simulink model "LQR_finished"  (R2018b)
settings: Solver=VariableStepAuto  StartTime=0.0  StopTime=25  MinStep=1e-100  RelTol=1e-3
model workspace (MAT data in the model file):
  Af = 0.027
  Cd = 32.3127
  Q = 1
  R = 1
  Rx = 1.6517
  Tf = 25
  g = 9.81
  height = 0.12
  m = 3
  rho = 1.225
  v = 0
  width = 0.25
values from neighbouring files (symbols this model uses):
  K = lqr(A,B,100,1)    [lab6.m]
  p = 1.225    [lab6.m]
settings Model: Creator=vallon2  LastModifiedBy=Sunny
settings SFSimCC: SimUseLocalCustomCode=off
settings RTWCC: RTWUseLocalCustomCode=off

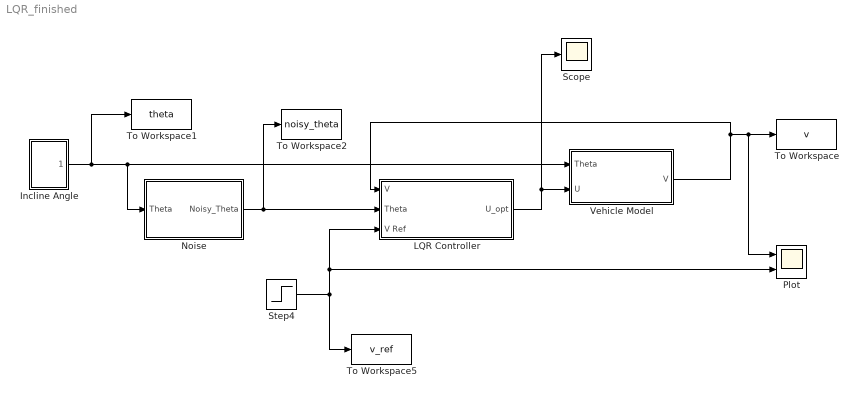
== system LQR_finished ==
  Incline Angle : Subsystem
  LQR Controller : Subsystem
  "Noise " : Subsystem
  "Plot " : Scope  NumInputPorts=2
  Scope : Scope
  Step4 : Step  Time=10  Before=0.5  SampleTime=0
  To Workspace : ToWorkspace  VariableName=v  SaveFormat=Timeseries  SampleTime=-1
  To Workspace1 : ToWorkspace  VariableName=theta  SaveFormat=Timeseries  SampleTime=-1
  To Workspace2 : ToWorkspace  VariableName=noisy_theta  SaveFormat=Timeseries  SampleTime=-1
  To Workspace5 : ToWorkspace  VariableName=v_ref  SaveFormat=Timeseries  SampleTime=-1
  Vehicle Model : Subsystem
  wires:
  Step4/1 -> To Workspace5/1, "Plot "/2, LQR Controller/3(V Ref)
  Vehicle Model/1(V) -> To Workspace/1, "Plot "/1, LQR Controller/1("V ")
  LQR Controller/1("U_opt ") -> Scope/1, Vehicle Model/2(U)
  "Noise "/1("Noisy_Theta ") -> LQR Controller/2(Theta), To Workspace2/1
  Incline Angle/1("Theta ") -> To Workspace1/1, Vehicle Model/1(Theta), "Noise "/1("Theta ")

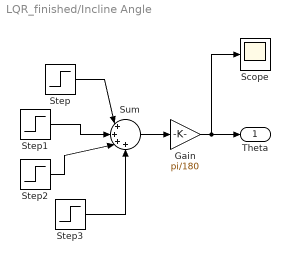
== system LQR_finished/Incline Angle ==
  Gain : Gain  Gain=pi/180
  Scope : Scope
  Step : Step  Time=3  After=10  SampleTime=0
  Step1 : Step  Time=8  After=10  SampleTime=0
  Step2 : Step  Time=13  After=-35  SampleTime=0
  Step3 : Step  Time=17  After=15  SampleTime=0
  Sum : Sum  Inputs=|++++
  "Theta " : Outport
  wires:
  Step/1 -> Sum/1
  Step1/1 -> Sum/2
  Step3/1 -> Sum/4
  Sum/1 -> Gain/1
  Gain/1 -> Scope/1, "Theta "/1
  Step2/1 -> Sum/3

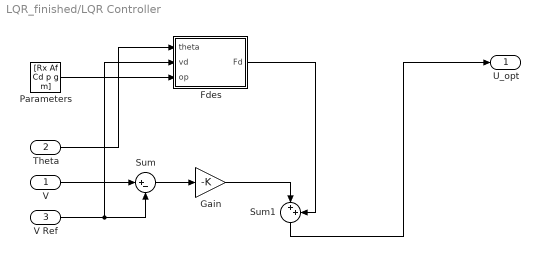
== system LQR_finished/LQR Controller ==
  "V " : Inport
  Theta : Inport  Port=2
  V Ref : Inport  Port=3
  Fdes : MATLAB Function  TreatAsAtomicUnit=on
  Gain : Gain  Gain=-K
  Parameters : Constant  Value=[Rx Af Cd p g m]
  Sum : Sum  Inputs=|+-
  Sum1 : Sum  Inputs=|++
  "U_opt " : Outport
  wires:
  "V "/1 -> Sum/1
  V Ref/1 -> Sum/2, Fdes/2(vd)
  Sum/1 -> Gain/1
  Fdes/1(Fd) -> Sum1/2
  Theta/1 -> Fdes/1(theta)
  Gain/1 -> Sum1/1
  Sum1/1 -> "U_opt "/1
  Parameters/1 -> Fdes/3(op)

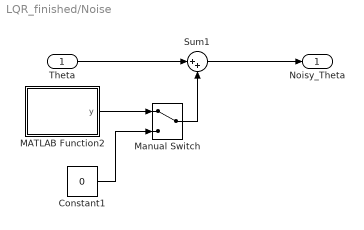
== system LQR_finished/Noise  ==
  "Theta " : Inport
  Constant1 : Constant  Value=0
  MATLAB Function2 : MATLAB Function  TreatAsAtomicUnit=on
  Manual Switch : ManualSwitch
  Sum1 : Sum  Inputs=|++
  "Noisy_Theta " : Outport
  wires:
  Constant1/1 -> Manual Switch/2
  Sum1/1 -> "Noisy_Theta "/1
  MATLAB Function2/1(y) -> Manual Switch/1
  "Theta "/1 -> Sum1/1
  Manual Switch/1 -> Sum1/2

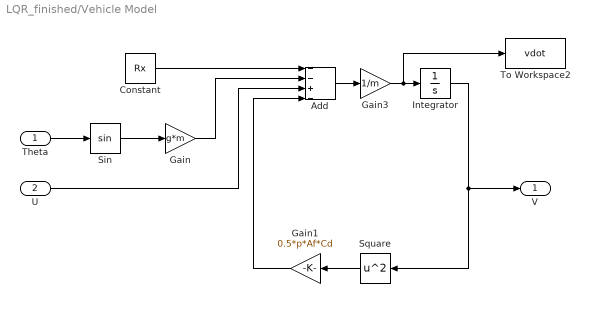
== system LQR_finished/Vehicle Model ==
  Theta : Inport
  U : Inport  Port=2
  Add : Sum  Inputs=--+-
  Constant : Constant  Value=Rx
  Gain : Gain  Gain=g*m
  Gain1 : Gain  Gain=0.5*p*Af*Cd
  Gain3 : Gain  Gain=1/m
  Integrator : Integrator
  Sin : Trigonometry
  Square : Math  Operator=square  SaturateOnIntegerOverflow=on
  To Workspace2 : ToWorkspace  VariableName=vdot  SaveFormat=Timeseries  SampleTime=-1
  V : Outport
  wires:
  Constant/1 -> Add/1
  Theta/1 -> Sin/1
  Sin/1 -> Gain/1
  Gain/1 -> Add/2
  U/1 -> Add/3
  Add/1 -> Gain3/1
  Square/1 -> Gain1/1
  Gain1/1 -> Add/4
  Integrator/1 -> Square/1, V/1
  Gain3/1 -> To Workspace2/1, Integrator/1

== matlab function LQR_finished/LQR Controller/Fdes ==
  data: theta input; Fd output; vd input; op input
function Fd = fcn( theta, vd, op)
Rx = op(1);
Af = op(2);
Cd = op(3);
p = op(4);
g = op(5);
m = op(6);
Fd = Rx+m*g*sin(theta)+0.5*p*Af*Cd*vd^2;

== matlab function LQR_finished/Noise /MATLAB Function2 ==
  data: y output
function y = noise
y = 0.01*randn(1);
